simulink model "moblienode_energy"  (R2018a)
settings: Solver=VariableStepAuto  StartTime=0.0  StopTime=10.0  RelTol=1e-3
libraries: dspmathops x4
settings Model: Creator=janish  LastModifiedBy=janish

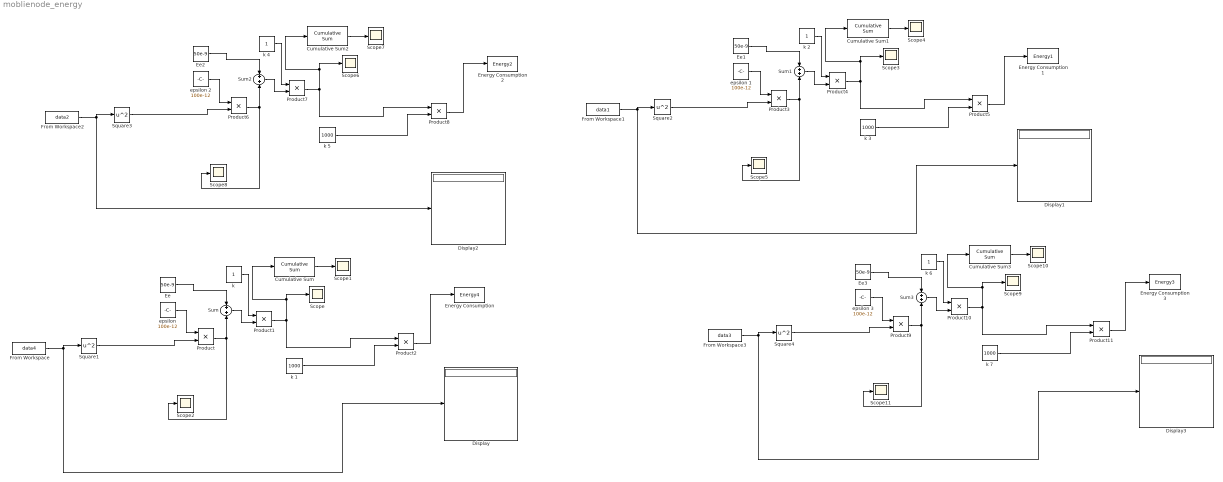
== system moblienode_energy ==
  Cumulative Sum{,1..3} (4 alike) : dspmathops/Cumulative Sum  dim=Channels (running sum)  InputProcessing=Columns as channels (frame based)  reset_popup=None  roundingMode=Floor  overflowMode=off  outputDataTypeStr=Inherit: Same as accumulator  outputMin=[]  outputMax=[]  outputLastDataTypeStr=Inherit: Same as accumulator
      settings: SourceProductName=DSP System Toolbox
  Display{,1..3} (4 alike) : Display
  Ee{,1..3} (4 alike) : Constant  Value=50e-9
  "Energy Consumption " : ToWorkspace  VariableName=Energy4  SampleTime=12060
      settings: MaxDataPoints=1
  Energy Consumption 1 : ToWorkspace  VariableName=Energy1  SampleTime=12060
      settings: MaxDataPoints=1
  Energy Consumption 2 : ToWorkspace  VariableName=Energy2  SampleTime=12060
      settings: MaxDataPoints=1
  Energy Consumption 3 : ToWorkspace  VariableName=Energy3  SampleTime=12060
      settings: MaxDataPoints=1
  From Workspace : FromWorkspace  VariableName=data4  SampleTime=12000
  From Workspace1 : FromWorkspace  VariableName=data1  SampleTime=12000
  From Workspace2 : FromWorkspace  VariableName=data2  SampleTime=12000
  From Workspace3 : FromWorkspace  VariableName=data3  SampleTime=12000
  Product{,1..11} (12 alike) : Product
  Scope{,1..11} (12 alike) : Scope
  Square{1..4} (4 alike) : Math  Operator=square  SaturateOnIntegerOverflow=on
  Sum{,1..3} (4 alike) : Sum
  epsilon {,1..3} (4 alike) : Constant  Value=100e-12
  k {,2,4,6} (4 alike) : Constant
  k {1,3,5,7} (4 alike) : Constant  Value=1000
  wires:
  From Workspace/1 -> Square1/1, Display/1
  Ee/1 -> Sum/1
  k 1/1 -> Product2/2
  Cumulative Sum/1 -> Scope1/1
  "k "/1 -> Product1/1
  "epsilon "/1 -> Product/1
  Product/1 -> Scope2/1, Sum/2
  Product1/1 -> Product2/1, Scope/1, Cumulative Sum/1
  Sum/1 -> Product1/2
  Product2/1 -> "Energy Consumption "/1
  Square1/1 -> Product/2
  From Workspace1/1 -> Square2/1, Display1/1
  Ee1/1 -> Sum1/1
  k 3/1 -> Product5/2
  Cumulative Sum1/1 -> Scope4/1
  k 2/1 -> Product4/1
  epsilon 1/1 -> Product3/1
  Product3/1 -> Scope5/1, Sum1/2
  Product4/1 -> Product5/1, Scope3/1, Cumulative Sum1/1
  Sum1/1 -> Product4/2
  Product5/1 -> Energy Consumption 1/1
  Square2/1 -> Product3/2
  From Workspace2/1 -> Square3/1, Display2/1
  Ee2/1 -> Sum2/1
  k 5/1 -> Product8/2
  Cumulative Sum2/1 -> Scope7/1
  k 4/1 -> Product7/1
  epsilon 2/1 -> Product6/1
  Product6/1 -> Scope8/1, Sum2/2
  Product7/1 -> Product8/1, Scope6/1, Cumulative Sum2/1
  Sum2/1 -> Product7/2
  Product8/1 -> Energy Consumption 2/1
  Square3/1 -> Product6/2
  From Workspace3/1 -> Square4/1, Display3/1
  Ee3/1 -> Sum3/1
  k 7/1 -> Product11/2
  Cumulative Sum3/1 -> Scope10/1
  k 6/1 -> Product10/1
  epsilon 3/1 -> Product9/1
  Product9/1 -> Scope11/1, Sum3/2
  Product10/1 -> Product11/1, Scope9/1, Cumulative Sum3/1
  Sum3/1 -> Product10/2
  Product11/1 -> Energy Consumption 3/1
  Square4/1 -> Product9/2
